simulink model "kopter_se_zavazim_simulace_2024a"  (R2024a)
settings: Solver=FixedStepAuto  StartTime=0.0  StopTime=5  FixedStep=0.01  RelTol=1e-3
values from neighbouring files (symbols this model uses):
  b_moment = 5.4e-6    (= 5.4e-06)    [parametry_kopter_se_zavazim.m]
  d = 1    [parametry_kopter_se_zavazim.m]
  g = 9.81    [parametry_kopter_se_zavazim.m]
  Ip = m*d^2    (= 1)    [parametry_kopter_se_zavazim.m]
  Ixx = 0.0222    [parametry_kopter_se_zavazim.m]
  Iyy = 0.0222    [parametry_kopter_se_zavazim.m]
  Izz = 0.0429    [parametry_kopter_se_zavazim.m]
  k_thrust = 2.3e-3    (= 0.0023)    [parametry_kopter_se_zavazim.m]
  M = 2    [parametry_kopter_se_zavazim.m]
  m = 1    [parametry_kopter_se_zavazim.m]
  Us_p = [(M+m)*g; 0; 0; 0]    [parametry_kopter_se_zavazim.m]
  Xinit_matrix = [xyz_init; uhly_init; zavazi_init]    [parametry_kopter_se_zavazim.m]
  Xinit_ss = [Xinit_matrix; [0 0 0 0 0 0 0 0]']    [parametry_kopter_se_zavazim.m]
  Xs_p = [0;0;0; 0;0;0; 0;0; 0;0;0; 0;0;0; 0;0]    [parametry_kopter_se_zavazim.m]
undefined symbols (not defined in the file or in its folder): L
libraries: simulink_extras x6
(part 2 of 5)

== matlab function kopter_se_zavazim_simulace_2024a/Nelinearni State-Space (se zavazim)/B ==
  data: roll input; B output; pitch input; yaw input; alpha input; beta input; M parameter; Ixx parameter; Iyy parameter; Izz parameter; Ip parameter; d parameter; m parameter
function B = fcn(roll, pitch, yaw, alpha, beta, M, Ixx, Iyy, Izz, Ip, d, m)
% Matice vstupu do soustavy kvadrokoptery se zavazim

phi_t = roll;
theta_t = pitch;
psi_t = yaw;

alpha_t = alpha;
beta_t = beta;

B = [ 
                                                                                                                                                                                                                                                                                                                                                                                                                                                                                                                                                                                                                                                                                                                                                                                                                                                                                                                                                                                                                                                                                                                                                                                                                                                                                                                                                                                                                                                                                                                                                                                                                                                                                                                                                                                                                                                                                                                                                                                                                                                                                                                                                                                                                                                                                                                                                                                                                                                                                                                                                                                                                                                                                                                                                                                                                                                                                                                                                                                                                                                                                                                                                                                                                                                                                                                                                                                                                                                                                                                                                                                                                                                                                                                                                                                                                                                                                                                                                                                                                                                                                                                                                                                                                                                                                                                                                                                                                                                                                                                                                                                                                                                                                                                                                                                                                                                                                                                                                                                                                                                          0,                                                                                                                                                                                                                                                                                                                                                                                                                                                                                                                                                   0,                                                                                                                                                                                                                                0,                                                                                                                                                                                                                                           0;
                                                                                                                                                                                                                                                                                                                                                                                                                                                                                                                                                                                                                                                                                                                                                                                                                                                                                                                                                                                                                                                                                                                                                                                                                                                                                                                                                                                                                                                                                                                                                                                                                                                                                                                                                                                                                                                                                                                                                                                                                                                                                                                                                                                                                                                                                                                                                                                                                                                                                                                                                                                                                                                                                                                                                                                                                                                                                                                                                                                                                                                                                                                                                                                                                                                                                                                                                                                                                                                                                                                                                                                                                                                                                                                                                                                                                                                                                                                                                                                                                                                                                                                                                                                                                                                                                                                                                                                                                                                                                                                                                                                                                                                                                                                                                                                                                                                                                                                                                                                                                                                          0,                                                                                                                                                                                                                                                                                                                                                                                                                                                                                                                                                   0,                                                                                                                                                                                                                                0,                                                                                                                                                                                                                                           0;
                                                                                                                                                                                                                                                                                                                                                                                                                                                                                                                                                                                                                                                                                                                                                                                                                                                                                                                                                                                                                                                                                                                                                                                                                                                                                                                                                                                                                                                                                                                                                                                                                                                                                                                                                                                                                                                                                                                                                                                                                                                                                                                                                                                                                                                                                                                                                                                                                                                                                                                                                                                                                                                                                                                                                                                                                                                                                                                                                                                                                                                                                                                                                                                                                                                                                                                                                                                                                                                                                                                                                                                                                                                                                                                                                                                                                                                                                                                                                                                                                                                                                                                                                                                                                                                                                                                                                                                                                                                                                                                                                                                                                                                                                                                                                                                                                                                                                                                                                                                                                                                          0,                                                                                                                                                                                                                                                                                                                                                                                                                                                                                                                                                   0,                                                                                                                                                                                                                                0,                                                                                                                                                                                                                                           0;
                                                                                                                                                                                                                                                                                                                                                                                                                                                                                                                                                                                                                                                                                                                                                                                                                                                                                                                                                                                                                                                                                                                                                                                                                                                                                                                                                                                                                                                                                                                                                                                                                                                                                                                                                                                                                                                                                                                                                                                                                                                                                                                                                                                                                                                                                                                                                                                                                                                                                                                                                                                                                                                                                                                                                                                                                                                                                                                                                                                                                                                                                                                                                                                                                                                                                                                                                                                                                                                                                                                                                                                                                                                                                                                                                                                                                                                                                                                                                                                                                                                                                                                                                                                                                                                                                                                                                                                                                                                                                                                                                                                                                                                                                                                                                                                                                                                                                                                                                                                                                                                          0,                                                                                                                                                                                                                                                                                                                                                                                                                                                                                                                                                   0,                                                                                                                                                                                                                                0,                                                                                                                                                                                                                                           0;
                                                                                                                                                                                                                                                                                                                                                                                                                                                                                                                                                                                                                                                                                                                                                                                                                                                                                                                                                                                                                                                                                                                                                                                                                                                                                                                                                                                                                                                                                                                                                                                                                                                                                                                                                                                                                                                                                                                                                                                                                                                                                                                                                                                                                                                                                                                                                                                                                                                                                                                                                                                                                                                                                                                                                                                                                                                                                                                                                                                                                                                                                                                                                                                                                                                                                                                                                                                                                                                                                                                                                                                                                                                                                                                                                                                                                                                                                                                                                                                                                                                                                                                                                                                                                                                                                                                                                                                                                                                                                                                                                                                                                                                                                                                                                                                                                                                                                                                                                                                                                                                          0,                                                                                                                                                                                                                                                                                                                                                                                                                                                                                                                                                   0,                                                                                                                                                                                                                                0,                                                                                                                                                                                                                                           0;
                                                                                                                                                                                                                                                                                                                                                                                                                                                                                                                                                                                                                                                                                                                                                                                                                                                                                                                                                                                                                                                                                                                                                                                                                                                                                                                                                                                                                                                                                                                                                                                                                                                                                                                                                                                                                                                                                                                                                                                                                                                                                                                                                                                                                                                                                                                                                                                                                                                                                                                                                                                                                                                                                                                                                                                                                                                                                                                                                                                                                                                                                                                                                                                                                                                                                                                                                                                                                                                                                                                                                                                                                                                                                                                                                                                                                                                                                                                                                                                                                                                                                                                                                                                                                                                                                                                                                                                                                                                                                                                                                                                                                                                                                                                                                                                                                                                                                                                                                                                                                                                          0,                                                                                                                                                                                                                                                                                                                                                                                                                                                                                                                                                   0,                                                                                                                                                                                                                                0,                                                                                                                                                                                                                                           0;
                                                                                                                                                                                                                                                                                                                                                                                                                                                                                                                                                                                                                                                                                                                                                                                                                                                                                                                                                                                                                                                                                                                                                                                                                                                                                                                                                                                                                                                                                                                                                                                                                                                                                                                                                                                                                                                                                                                                                                                                                                                                                                                                                                                                                                                                                                                                                                                                                                                                                                                                                                                                                                                                                                                                                                                                                                                                                                                                                                                                                                                                                                                                                                                                                                                                                                                                                                                                                                                                                                                                                                                                                                                                                                                                                                                                                                                                                                                                                                                                                                                                                                                                                                                                                                                                                                                                                                                                                                                                                                                                                                                                                                                                                                                                                                                                                                                                                                                                                                                                                                                          0,                                                                                                                                                                                                                                                                                                                                                                                                                                                                                                                                                   0,                                                                                                                                                                                                                                0,                                                                                                                                                                                                                                           0;
                                                                                                                                                                                                                                                                                                                                                                                                                                                                                                                                                                                                                                                                                                                                                                                                                                                                                                                                                                                                                                                                                                                                                                                                                                                                                                                                                                                                                                                                                                                                                                                                                                                                                                                                                                                                                                                                                                                                                                                                                                                                                                                                                                                                                                                                                                                                                                                                                                                                                                                                                                                                                                                                                                                                                                                                                                                                                                                                                                                                                                                                                                                                                                                                                                                                                                                                                                                                                                                                                                                                                                                                                                                                                                                                                                                                                                                                                                                                                                                                                                                                                                                                                                                                                                                                                                                                                                                                                                                                                                                                                                                                                                                                                                                                                                                                                                                                                                                                                                                                                                                          0,                                                                                                                                                                                                                                                                                                                                                                                                                                                                                                                                                   0,                                                                                                                                                                                                                                0,                                                                                                                                                                                                                                           0;
(Ip^2*M^2*sin(phi_t)*sin(psi_t) + Ip^2*m^2*sin(phi_t)*sin(psi_t) + Ip*d^2*m^3*sin(phi_t)*sin(psi_t) + Ip^2*M^2*cos(phi_t)*cos(psi_t)*sin(theta_t) + Ip^2*m^2*cos(phi_t)*cos(psi_t)*sin(theta_t) + 2*Ip^2*M*m*sin(phi_t)*sin(psi_t) + d^4*m^4*sin(alpha_t)^2*sin(phi_t)*sin(psi_t) - d^4*m^4*sin(alpha_t)^4*sin(phi_t)*sin(psi_t) - d^4*m^4*cos(beta_t)^2*sin(alpha_t)^2*sin(phi_t)*sin(psi_t) + d^4*m^4*cos(beta_t)^2*sin(alpha_t)^4*sin(phi_t)*sin(psi_t) + 2*M*d^4*m^3*sin(alpha_t)^2*sin(phi_t)*sin(psi_t) - M*d^4*m^3*sin(alpha_t)^4*sin(phi_t)*sin(psi_t) + 2*Ip*M*d^2*m^2*sin(phi_t)*sin(psi_t) + Ip*M^2*d^2*m*sin(phi_t)*sin(psi_t) + 2*Ip^2*M*m*cos(phi_t)*cos(psi_t)*sin(theta_t) + M^2*d^4*m^2*sin(alpha_t)^2*sin(phi_t)*sin(psi_t) + d^4*m^4*cos(phi_t)*cos(psi_t)*sin(alpha_t)^2*sin(theta_t) - d^4*m^4*cos(phi_t)*cos(psi_t)*sin(alpha_t)^4*sin(theta_t) + Ip*d^2*m^3*cos(phi_t)*cos(psi_t)*sin(theta_t) + 2*M*d^4*m^3*cos(phi_t)*cos(psi_t)*sin(alpha_t)^2*sin(theta_t) - M*d^4*m^3*cos(phi_t)*cos(psi_t)*sin(alpha_t)^4*sin(theta_t) + 2*Ip*M*d^2*m^2*cos(phi_t)*cos(psi_t)*sin(theta_t) + Ip*M^2*d^2*m*cos(phi_t)*cos(psi_t)*sin(theta_t) - d^4*m^4*cos(alpha_t)^2*sin(alpha_t)^2*sin(beta_t)^2*sin(phi_t)*sin(psi_t) + d^4*m^4*cos(alpha_t)*cos(beta_t)*cos(phi_t)*sin(alpha_t)^3*cos(theta_t) - Ip*d^2*m^3*cos(alpha_t)^2*sin(beta_t)^2*sin(phi_t)*sin(psi_t) - Ip*d^2*m^3*cos(beta_t)^2*sin(alpha_t)^2*sin(phi_t)*sin(psi_t) - M*d^4*m^3*cos(beta_t)^2*sin(alpha_t)^2*sin(phi_t)*sin(psi_t) + M^2*d^4*m^2*cos(phi_t)*cos(psi_t)*sin(alpha_t)^2*sin(theta_t) + d^4*m^4*cos(beta_t)*cos(psi_t)*sin(alpha_t)^2*sin(beta_t)*sin(phi_t) - d^4*m^4*cos(beta_t)*cos(psi_t)*sin(alpha_t)^4*sin(beta_t)*sin(phi_t) + Ip*M*d^2*m^2*sin(alpha_t)^2*sin(phi_t)*sin(psi_t) + Ip*M^2*d^2*m*sin(alpha_t)^2*sin(phi_t)*sin(psi_t) - d^4*m^4*cos(alpha_t)*cos(beta_t)^3*cos(phi_t)*sin(alpha_t)^3*cos(theta_t) - d^4*m^4*cos(beta_t)^2*cos(phi_t)*cos(psi_t)*sin(alpha_t)^2*sin(theta_t) + d^4*m^4*cos(beta_t)^2*cos(phi_t)*cos(psi_t)*sin(alpha_t)^4*sin(theta_t) - d^4*m^4*cos(alpha_t)^2*cos(phi_t)*cos(psi_t)*sin(alpha_t)^2*sin(beta_t)^2*sin(theta_t) - Ip*d^2*m^3*cos(alpha_t)^2*cos(phi_t)*cos(psi_t)*sin(beta_t)^2*sin(theta_t) - Ip*d^2*m^3*cos(beta_t)^2*cos(phi_t)*cos(psi_t)*sin(alpha_t)^2*sin(theta_t) - M*d^4*m^3*cos(beta_t)^2*cos(phi_t)*cos(psi_t)*sin(alpha_t)^2*sin(theta_t) + Ip*d^2*m^3*cos(alpha_t)*cos(beta_t)*cos(phi_t)*sin(alpha_t)*cos(theta_t) + Ip*M*d^2*m^2*cos(phi_t)*cos(psi_t)*sin(alpha_t)^2*sin(theta_t) + Ip*M^2*d^2*m*cos(phi_t)*cos(psi_t)*sin(alpha_t)^2*sin(theta_t) - d^4*m^4*cos(beta_t)*cos(phi_t)*sin(alpha_t)^2*sin(beta_t)*sin(psi_t)*sin(theta_t) + d^4*m^4*cos(beta_t)*cos(phi_t)*sin(alpha_t)^4*sin(beta_t)*sin(psi_t)*sin(theta_t) - d^4*m^4*cos(alpha_t)*cos(beta_t)*cos(phi_t)*sin(alpha_t)^3*sin(beta_t)^2*cos(theta_t) - M*d^4*m^3*cos(alpha_t)^2*sin(alpha_t)^2*sin(beta_t)^2*sin(phi_t)*sin(psi_t) - d^4*m^4*cos(alpha_t)^2*cos(beta_t)*cos(psi_t)*sin(alpha_t)^2*sin(beta_t)*sin(phi_t) + M*d^4*m^3*cos(alpha_t)*cos(beta_t)*cos(phi_t)*sin(alpha_t)^3*cos(theta_t) - Ip*M*d^2*m^2*cos(alpha_t)^2*sin(beta_t)^2*sin(phi_t)*sin(psi_t) - Ip*M*d^2*m^2*cos(beta_t)^2*sin(alpha_t)^2*sin(phi_t)*sin(psi_t) - Ip*d^2*m^3*cos(alpha_t)^2*cos(beta_t)*cos(psi_t)*sin(beta_t)*sin(phi_t) + Ip*d^2*m^3*cos(beta_t)*cos(psi_t)*sin(alpha_t)^2*sin(beta_t)*sin(phi_t) + M*d^4*m^3*cos(beta_t)*cos(psi_t)*sin(alpha_t)^2*sin(beta_t)*sin(phi_t) + Ip*M*d^2*m^2*cos(beta_t)*cos(psi_t)*sin(alpha_t)^2*sin(beta_t)*sin(phi_t) - M*d^4*m^3*cos(alpha_t)^2*cos(phi_t)*cos(psi_t)*sin(alpha_t)^2*sin(beta_t)^2*sin(theta_t) - Ip*M*d^2*m^2*cos(alpha_t)^2*cos(phi_t)*cos(psi_t)*sin(beta_t)^2*sin(theta_t) - Ip*M*d^2*m^2*cos(beta_t)^2*cos(phi_t)*cos(psi_t)*sin(alpha_t)^2*sin(theta_t) + d^4*m^4*cos(alpha_t)^2*cos(beta_t)*cos(phi_t)*sin(alpha_t)^2*sin(beta_t)*sin(psi_t)*sin(theta_t) + Ip*M*d^2*m^2*cos(alpha_t)*cos(beta_t)*cos(phi_t)*sin(alpha_t)*cos(theta_t) + Ip*d^2*m^3*cos(alpha_t)^2*cos(beta_t)*cos(phi_t)*sin(beta_t)*sin(psi_t)*sin(theta_t) - Ip*d^2*m^3*cos(beta_t)*cos(phi_t)*sin(alpha_t)^2*sin(beta_t)*sin(psi_t)*sin(theta_t) - M*d^4*m^3*cos(beta_t)*cos(phi_t)*sin(alpha_t)^2*sin(beta_t)*sin(psi_t)*sin(theta_t) - M*d^4*m^3*cos(alpha_t)^2*cos(beta_t)*cos(psi_t)*sin(alpha_t)^2*sin(beta_t)*sin(phi_t) - Ip*M*d^2*m^2*cos(alpha_t)^2*cos(beta_t)*cos(psi_t)*sin(beta_t)*sin(phi_t) + M*d^4*m^3*cos(alpha_t)^2*cos(beta_t)*cos(phi_t)*sin(alpha_t)^2*sin(beta_t)*sin(psi_t)*sin(theta_t) + Ip*M*d^2*m^2*cos(alpha_t)^2*cos(beta_t)*cos(phi_t)*sin(beta_t)*sin(psi_t)*sin(theta_t) - Ip*M*d^2*m^2*cos(beta_t)*cos(phi_t)*sin(alpha_t)^2*sin(beta_t)*sin(psi_t)*sin(theta_t))/((M + m)*(- d^2*m^2*cos(beta_t)^2*sin(alpha_t)^2 - d^2*m^2*sin(alpha_t)^2*sin(beta_t)^2 + d^2*m^2*sin(alpha_t)^2 + M*d^2*m*sin(alpha_t)^2 + Ip*m + Ip*M)*(- d^2*m^2*cos(alpha_t)^2*cos(beta_t)^2 - d^2*m^2*cos(alpha_t)^2*sin(beta_t)^2 - d^2*m^2*sin(alpha_t)^2 + d^2*m^2 + M*d^2*m + Ip*m + Ip*M)),                                                                                                                                                                                                                                                                                                                                                                                                                                                                                                                                                   0,                                                                                                                                                                                                                                0,                                                                                                                                                                                                                                           0;
(Ip^2*M^2*cos(phi_t)*sin(psi_t)*sin(theta_t) - Ip^2*m^2*cos(psi_t)*sin(phi_t) - Ip^2*M^2*cos(psi_t)*sin(phi_t) + Ip^2*m^2*cos(phi_t)*sin(psi_t)*sin(theta_t) - 2*Ip^2*M*m*cos(psi_t)*sin(phi_t) - d^4*m^4*cos(psi_t)*sin(alpha_t)^2*sin(phi_t) + d^4*m^4*cos(psi_t)*sin(alpha_t)^4*sin(phi_t) - Ip*d^2*m^3*cos(psi_t)*sin(phi_t) + d^4*m^4*cos(psi_t)*sin(alpha_t)^2*sin(beta_t)^2*sin(phi_t) - d^4*m^4*cos(psi_t)*sin(alpha_t)^4*sin(beta_t)^2*sin(phi_t) - 2*M*d^4*m^3*cos(psi_t)*sin(alpha_t)^2*sin(phi_t) + M*d^4*m^3*cos(psi_t)*sin(alpha_t)^4*sin(phi_t) - 2*Ip*M*d^2*m^2*cos(psi_t)*sin(phi_t) - Ip*M^2*d^2*m*cos(psi_t)*sin(phi_t) + 2*Ip^2*M*m*cos(phi_t)*sin(psi_t)*sin(theta_t) - M^2*d^4*m^2*cos(psi_t)*sin(alpha_t)^2*sin(phi_t) + d^4*m^4*cos(phi_t)*sin(alpha_t)^2*sin(psi_t)*sin(theta_t) - d^4*m^4*cos(phi_t)*sin(alpha_t)^4*sin(psi_t)*sin(theta_t) + Ip*d^2*m^3*cos(phi_t)*sin(psi_t)*sin(theta_t) + 2*M*d^4*m^3*cos(phi_t)*sin(alpha_t)^2*sin(psi_t)*sin(theta_t) - M*d^4*m^3*cos(phi_t)*sin(alpha_t)^4*sin(psi_t)*sin(theta_t) + d^4*m^4*cos(alpha_t)^2*cos(beta_t)^2*cos(psi_t)*sin(alpha_t)^2*sin(phi_t) + 2*Ip*M*d^2*m^2*cos(phi_t)*sin(psi_t)*sin(theta_t) + Ip*M^2*d^2*m*cos(phi_t)*sin(psi_t)*sin(theta_t) + Ip*d^2*m^3*cos(alpha_t)^2*cos(beta_t)^2*cos(psi_t)*sin(phi_t) + Ip*d^2*m^3*cos(psi_t)*sin(alpha_t)^2*sin(beta_t)^2*sin(phi_t) + M*d^4*m^3*cos(psi_t)*sin(alpha_t)^2*sin(beta_t)^2*sin(phi_t) + d^4*m^4*cos(alpha_t)*cos(phi_t)*sin(alpha_t)^3*sin(beta_t)*cos(theta_t) + M^2*d^4*m^2*cos(phi_t)*sin(alpha_t)^2*sin(psi_t)*sin(theta_t) - Ip*M*d^2*m^2*cos(psi_t)*sin(alpha_t)^2*sin(phi_t) - Ip*M^2*d^2*m*cos(psi_t)*sin(alpha_t)^2*sin(phi_t) - d^4*m^4*cos(beta_t)*sin(alpha_t)^2*sin(beta_t)*sin(phi_t)*sin(psi_t) + d^4*m^4*cos(beta_t)*sin(alpha_t)^4*sin(beta_t)*sin(phi_t)*sin(psi_t) - d^4*m^4*cos(alpha_t)*cos(phi_t)*sin(alpha_t)^3*sin(beta_t)^3*cos(theta_t) - d^4*m^4*cos(phi_t)*sin(alpha_t)^2*sin(beta_t)^2*sin(psi_t)*sin(theta_t) + d^4*m^4*cos(phi_t)*sin(alpha_t)^4*sin(beta_t)^2*sin(psi_t)*sin(theta_t) - d^4*m^4*cos(alpha_t)^2*cos(beta_t)^2*cos(phi_t)*sin(alpha_t)^2*sin(psi_t)*sin(theta_t) - Ip*d^2*m^3*cos(alpha_t)^2*cos(beta_t)^2*cos(phi_t)*sin(psi_t)*sin(theta_t) - Ip*d^2*m^3*cos(phi_t)*sin(alpha_t)^2*sin(beta_t)^2*sin(psi_t)*sin(theta_t) - M*d^4*m^3*cos(phi_t)*sin(alpha_t)^2*sin(beta_t)^2*sin(psi_t)*sin(theta_t) - d^4*m^4*cos(beta_t)*cos(phi_t)*cos(psi_t)*sin(alpha_t)^2*sin(beta_t)*sin(theta_t) + d^4*m^4*cos(beta_t)*cos(phi_t)*cos(psi_t)*sin(alpha_t)^4*sin(beta_t)*sin(theta_t) + Ip*d^2*m^3*cos(alpha_t)*cos(phi_t)*sin(alpha_t)*sin(beta_t)*cos(theta_t) + Ip*M*d^2*m^2*cos(phi_t)*sin(alpha_t)^2*sin(psi_t)*sin(theta_t) + Ip*M^2*d^2*m*cos(phi_t)*sin(alpha_t)^2*sin(psi_t)*sin(theta_t) + M*d^4*m^3*cos(alpha_t)^2*cos(beta_t)^2*cos(psi_t)*sin(alpha_t)^2*sin(phi_t) + Ip*M*d^2*m^2*cos(alpha_t)^2*cos(beta_t)^2*cos(psi_t)*sin(phi_t) - d^4*m^4*cos(alpha_t)*cos(beta_t)^2*cos(phi_t)*sin(alpha_t)^3*sin(beta_t)*cos(theta_t) + Ip*M*d^2*m^2*cos(psi_t)*sin(alpha_t)^2*sin(beta_t)^2*sin(phi_t) + d^4*m^4*cos(alpha_t)^2*cos(beta_t)*sin(alpha_t)^2*sin(beta_t)*sin(phi_t)*sin(psi_t) + M*d^4*m^3*cos(alpha_t)*cos(phi_t)*sin(alpha_t)^3*sin(beta_t)*cos(theta_t) + Ip*d^2*m^3*cos(alpha_t)^2*cos(beta_t)*sin(beta_t)*sin(phi_t)*sin(psi_t) - Ip*d^2*m^3*cos(beta_t)*sin(alpha_t)^2*sin(beta_t)*sin(phi_t)*sin(psi_t) - M*d^4*m^3*cos(beta_t)*sin(alpha_t)^2*sin(beta_t)*sin(phi_t)*sin(psi_t) + Ip*M*d^2*m^2*cos(alpha_t)^2*cos(beta_t)*sin(beta_t)*sin(phi_t)*sin(psi_t) - Ip*M*d^2*m^2*cos(beta_t)*sin(alpha_t)^2*sin(beta_t)*sin(phi_t)*sin(psi_t) - M*d^4*m^3*cos(alpha_t)^2*cos(beta_t)^2*cos(phi_t)*sin(alpha_t)^2*sin(psi_t)*sin(theta_t) - Ip*M*d^2*m^2*cos(alpha_t)^2*cos(beta_t)^2*cos(phi_t)*sin(psi_t)*sin(theta_t) + d^4*m^4*cos(alpha_t)^2*cos(beta_t)*cos(phi_t)*cos(psi_t)*sin(alpha_t)^2*sin(beta_t)*sin(theta_t) + Ip*d^2*m^3*cos(alpha_t)^2*cos(beta_t)*cos(phi_t)*cos(psi_t)*sin(beta_t)*sin(theta_t) - Ip*M*d^2*m^2*cos(phi_t)*sin(alpha_t)^2*sin(beta_t)^2*sin(psi_t)*sin(theta_t) - Ip*d^2*m^3*cos(beta_t)*cos(phi_t)*cos(psi_t)*sin(alpha_t)^2*sin(beta_t)*sin(theta_t) - M*d^4*m^3*cos(beta_t)*cos(phi_t)*cos(psi_t)*sin(alpha_t)^2*sin(beta_t)*sin(theta_t) + Ip*M*d^2*m^2*cos(alpha_t)*cos(phi_t)*sin(alpha_t)*sin(beta_t)*cos(theta_t) + M*d^4*m^3*cos(alpha_t)^2*cos(beta_t)*sin(alpha_t)^2*sin(beta_t)*sin(phi_t)*sin(psi_t) + M*d^4*m^3*cos(alpha_t)^2*cos(beta_t)*cos(phi_t)*cos(psi_t)*sin(alpha_t)^2*sin(beta_t)*sin(theta_t) + Ip*M*d^2*m^2*cos(alpha_t)^2*cos(beta_t)*cos(phi_t)*cos(psi_t)*sin(beta_t)*sin(theta_t) - Ip*M*d^2*m^2*cos(beta_t)*cos(phi_t)*cos(psi_t)*sin(alpha_t)^2*sin(beta_t)*sin(theta_t))/((M + m)*(- d^2*m^2*cos(beta_t)^2*sin(alpha_t)^2 - d^2*m^2*sin(alpha_t)^2*sin(beta_t)^2 + d^2*m^2*sin(alpha_t)^2 + M*d^2*m*sin(alpha_t)^2 + Ip*m + Ip*M)*(- d^2*m^2*cos(alpha_t)^2*cos(beta_t)^2 - d^2*m^2*cos(alpha_t)^2*sin(beta_t)^2 - d^2*m^2*sin(alpha_t)^2 + d^2*m^2 + M*d^2*m + Ip*m + Ip*M)),                                                                                                                                                                                                                                                                                                                                                                                                                                                                                                                                                   0,                                                                                                                                                                                                                                0,                                                                                                                                                                                                                                           0;
                                                                                                                                                                                                                                                                                                                                                                                                                                                                                                                                                                                                                                                                                                                                                                                                                                                                                                                                                                                                                                                                                                                                                                                                                                                                                                                                                                                                                                                                                                                                                                                                                                                                                                                                                                                                                                                                                                                                                                                                                                                                                                                                                                                                                                                                                                                                                                                                                                                                                                                                                                                                                                                                                                                                                                                                                                                                                                                                                                                                                                                                                                                                                                                                                                                                                                                                                                                                                                                                                                                                                                                                                                                                                                                                                                                                                                                                                                                                                                                                                                                                                                                                                                                                                                                                                                                     (d^2*m^2*cos(phi_t)*cos(theta_t) + Ip*M*cos(phi_t)*cos(theta_t) + Ip*m*cos(phi_t)*cos(theta_t) + M*d^2*m*cos(phi_t)*cos(theta_t) - d^2*m^2*cos(alpha_t)^2*cos(beta_t)^2*cos(phi_t)*cos(theta_t) - d^2*m^2*cos(alpha_t)^2*cos(phi_t)*sin(beta_t)^2*cos(theta_t) + d^2*m^2*cos(alpha_t)*cos(beta_t)*sin(alpha_t)*sin(phi_t)*sin(psi_t) - d^2*m^2*cos(alpha_t)*cos(psi_t)*sin(alpha_t)*sin(beta_t)*sin(phi_t) + d^2*m^2*cos(alpha_t)*cos(beta_t)*cos(phi_t)*cos(psi_t)*sin(alpha_t)*sin(theta_t) + d^2*m^2*cos(alpha_t)*cos(phi_t)*sin(alpha_t)*sin(beta_t)*sin(psi_t)*sin(theta_t))/((M + m)*(- d^2*m^2*cos(alpha_t)^2*cos(beta_t)^2 - d^2*m^2*cos(alpha_t)^2*sin(beta_t)^2 - d^2*m^2*sin(alpha_t)^2 + d^2*m^2 + M*d^2*m + Ip*m + Ip*M)),                                                                                                                                                                                                                                                                                                                                                                                                                                                                                                                                                   0,                                                                                                                                                                                                                                0,                                                                                                                                                                                                                                           0;
                                                                                                                                                                                                                                                                                                                                                                                                                                                                                                                                                                                                                                                                                                                                                                                                                                                                                                                                                                                                                                                                                                                                                                                                                                                                                                                                                                                                                                                                                                                                                                                                                                                                                                                                                                                                                                                                                                                                                                                                                                                                                                                                                                                                                                                                                                                                                                                                                                                                                                                                                                                                                                                                                                                                                                                                                                                                                                                                                                                                                                                                                                                                                                                                                                                                                                                                                                                                                                                                                                                                                                                                                                                                                                                                                                                                                                                                                                                                                                                                                                                                                                                                                                                                                                                                                                                                                                                                                                                                                                                                                                                                                                                                                                                                                                                                                                                                                                                                                                                                                                                          0, (- Iyy^2*cos(phi_t)^2*cos(theta_t)^2*sin(phi_t)^2 - Iyy^2*cos(theta_t)^2*sin(phi_t)^4 + Iyy^2*cos(theta_t)^2*sin(phi_t)^2 + Izz*Iyy*cos(phi_t)^2*cos(theta_t)^2*sin(phi_t)^2 + Izz*Iyy*cos(phi_t)^2*cos(theta_t)^2 + Izz*Iyy*cos(theta_t)^2*sin(phi_t)^4 - Ixx*Iyy*sin(phi_t)^2*sin(theta_t)^2 + Ixx*Iyy*sin(theta_t)^2 + Ixx*Izz*sin(phi_t)^2*sin(theta_t)^2)/(Ixx*cos(theta_t)^2*(- Iyy^2*cos(phi_t)^2*sin(phi_t)^2 - Iyy^2*sin(phi_t)^4 + Iyy^2*sin(phi_t)^2 + Izz*Iyy*cos(phi_t)^2*sin(phi_t)^2 + Izz*Iyy*cos(phi_t)^2 + Izz*Iyy*sin(phi_t)^4)), -(cos(phi_t)*sin(phi_t)*sin(theta_t)*(Iyy - Izz))/(cos(theta_t)*(- Iyy^2*cos(phi_t)^2*sin(phi_t)^2 - Iyy^2*sin(phi_t)^4 + Iyy^2*sin(phi_t)^2 + Izz*Iyy*cos(phi_t)^2*sin(phi_t)^2 + Izz*Iyy*cos(phi_t)^2 + Izz*Iyy*sin(phi_t)^4)), (sin(theta_t)*(Iyy - Iyy*sin(phi_t)^2 + Izz*sin(phi_t)^2))/(cos(theta_t)^2*(- Iyy^2*cos(phi_t)^2*sin(phi_t)^2 - Iyy^2*sin(phi_t)^4 + Iyy^2*sin(phi_t)^2 + Izz*Iyy*cos(phi_t)^2*sin(phi_t)^2 + Izz*Iyy*cos(phi_t)^2 + Izz*Iyy*sin(phi_t)^4));
                                                                                                                                                                                                                                                                                                                                                                                                                                                                                                                                                                                                                                                                                                                                                                                                                                                                                                                                                                                                                                                                                                                                                                                                                                                                                                                                                                                                                                                                                                                                                                                                                                                                                                                                                                                                                                                                                                                                                                                                                                                                                                                                                                                                                                                                                                                                                                                                                                                                                                                                                                                                                                                                                                                                                                                                                                                                                                                                                                                                                                                                                                                                                                                                                                                                                                                                                                                                                                                                                                                                                                                                                                                                                                                                                                                                                                                                                                                                                                                                                                                                                                                                                                                                                                                                                                                                                                                                                                                                                                                                                                                                                                                                                                                                                                                                                                                                                                                                                                                                                                                          0,                                                                                                                                                                                                                                                                                                                    -(cos(phi_t)*sin(phi_t)*sin(theta_t)*(Iyy - Izz))/(cos(theta_t)*(- Iyy^2*cos(phi_t)^2*sin(phi_t)^2 - Iyy^2*sin(phi_t)^4 + Iyy^2*sin(phi_t)^2 + Izz*Iyy*cos(phi_t)^2*sin(phi_t)^2 + Izz*Iyy*cos(phi_t)^2 + Izz*Iyy*sin(phi_t)^4)),                            (Izz*cos(phi_t)^2 + Iyy*sin(phi_t)^2)/(- Iyy^2*cos(phi_t)^2*sin(phi_t)^2 - Iyy^2*sin(phi_t)^4 + Iyy^2*sin(phi_t)^2 + Izz*Iyy*cos(phi_t)^2*sin(phi_t)^2 + Izz*Iyy*cos(phi_t)^2 + Izz*Iyy*sin(phi_t)^4),                         -(cos(phi_t)*sin(phi_t)*(Iyy - Izz))/(cos(theta_t)*(- Iyy^2*cos(phi_t)^2*sin(phi_t)^2 - Iyy^2*sin(phi_t)^4 + Iyy^2*sin(phi_t)^2 + Izz*Iyy*cos(phi_t)^2*sin(phi_t)^2 + Izz*Iyy*cos(phi_t)^2 + Izz*Iyy*sin(phi_t)^4));
                                                                                                                                                                                                                                                                                                                                                                                                                                                                                                                                                                                                                                                                                                                                                                                                                                                                                                                                                                                                                                                                                                                                                                                                                                                                                                                                                                                                                                                                                                                                                                                                                                                                                                                                                                                                                                                                                                                                                                                                                                                                                                                                                                                                                                                                                                                                                                                                                                                                                                                                                                                                                                                                                                                                                                                                                                                                                                                                                                                                                                                                                                                                                                                                                                                                                                                                                                                                                                                                                                                                                                                                                                                                                                                                                                                                                                                                                                                                                                                                                                                                                                                                                                                                                                                                                                                                                                                                                                                                                                                                                                                                                                                                                                                                                                                                                                                                                                                                                                                                                                                          0,                                                                                                                                                                                                                                                                                                         (sin(theta_t)*(Iyy - Iyy*sin(phi_t)^2 + Izz*sin(phi_t)^2))/(cos(theta_t)^2*(- Iyy^2*cos(phi_t)^2*sin(phi_t)^2 - Iyy^2*sin(phi_t)^4 + Iyy^2*sin(phi_t)^2 + Izz*Iyy*cos(phi_t)^2*sin(phi_t)^2 + Izz*Iyy*cos(phi_t)^2 + Izz*Iyy*sin(phi_t)^4)),              -(cos(phi_t)*sin(phi_t)*(Iyy - Izz))/(cos(theta_t)*(- Iyy^2*cos(phi_t)^2*sin(phi_t)^2 - Iyy^2*sin(phi_t)^4 + Iyy^2*sin(phi_t)^2 + Izz*Iyy*cos(phi_t)^2*sin(phi_t)^2 + Izz*Iyy*cos(phi_t)^2 + Izz*Iyy*sin(phi_t)^4)),                (Iyy - Iyy*sin(phi_t)^2 + Izz*sin(phi_t)^2)/(cos(theta_t)^2*(- Iyy^2*cos(phi_t)^2*sin(phi_t)^2 - Iyy^2*sin(phi_t)^4 + Iyy^2*sin(phi_t)^2 + Izz*Iyy*cos(phi_t)^2*sin(phi_t)^2 + Izz*Iyy*cos(phi_t)^2 + Izz*Iyy*sin(phi_t)^4));
                                                                                                                                                                                                                                                                                                                                                                                                                                                                                                                                                                                                                                                                                                                                                                                                                                                                                                                                                                                                                                                                                                                                                                                                                                                                                                                                                                                                                                                                                                                                                                                                                                                                                                                                                                                                                                                                                                                                                                                                                                                                                                                                                                                                                                                                                                                                                                                                                                                                                                                                                                                                                                                                                                                                                                                                                                                                                                                                                                                                                                                                                                                                                                                                                                                                                                                                                                                                                                                                                                                                                                                                                                                                                                                                                                                                                                                                                                                                                                                                                                                                                                                                                                                                                                                                                                                                                                                                                                                                                                                                                                                                                       -(d*m*cos(phi_t)*sin(alpha_t)*cos(theta_t) + d*m*cos(alpha_t)*cos(beta_t)*sin(phi_t)*sin(psi_t) - d*m*cos(alpha_t)*cos(psi_t)*sin(beta_t)*sin(phi_t) + d*m*cos(alpha_t)*cos(beta_t)*cos(phi_t)*cos(psi_t)*sin(theta_t) + d*m*cos(alpha_t)*cos(phi_t)*sin(beta_t)*sin(psi_t)*sin(theta_t))/(- d^2*m^2*cos(alpha_t)^2*cos(beta_t)^2 - d^2*m^2*cos(alpha_t)^2*sin(beta_t)^2 - d^2*m^2*sin(alpha_t)^2 + d^2*m^2 + M*d^2*m + Ip*m + Ip*M),                                                                                                                                                                                                                                                                                                                                                                                                                                                                                                                                                   0,                                                                                                                                                                                                                                0,                                                                                                                                                                                                                                           0;
                                                                                                                                                                                                                                                                                                                                                                                                                                                                                                                                                                                                                                                                                                                                                                                                                                                                                                                                                                                                                                                                                                                                                                                                                                                                                                                                                                                                                                                                                                                                                                                                                                                                                                                                                                                                                                                                                                                                                                                                                                                                                                                                                                                                                                                                                                                                                                                                                                                                                                                                                                                                                                                                                                                                                                                                                                                                                                                                                                                                                                                                                                                                                                                                                                                                                                                                                                                                                                                                                                                                                                                                                                                                                                                                                                                                                                                                                                                                                                                                                                                                                                                                                                                                                                                                                                                                                                                                                                                                                                                                                                                                                                                              (d*m*cos(beta_t)*cos(psi_t)*sin(alpha_t)*sin(phi_t) + d*m*sin(alpha_t)*sin(beta_t)*sin(phi_t)*sin(psi_t) - d*m*cos(beta_t)*cos(phi_t)*sin(alpha_t)*sin(psi_t)*sin(theta_t) + d*m*cos(phi_t)*cos(psi_t)*sin(alpha_t)*sin(beta_t)*sin(theta_t))/(- d^2*m^2*cos(beta_t)^2*sin(alpha_t)^2 - d^2*m^2*sin(alpha_t)^2*sin(beta_t)^2 + d^2*m^2*sin(alpha_t)^2 + M*d^2*m*sin(alpha_t)^2 + Ip*m + Ip*M),                                                                                                                                                                                                                                                                                                                                                                                                                                                                                                                                                   0,                                                                                                                                                                                                                                0,                                                                                                                                                                                                                                           0];
